simulink library "wnnmodels"  (R2021b)
settings: Solver=VariableStepAuto  StartTime=0.0  StopTime=10.0  RelTol=1e-3
undefined symbols (not defined in the file or in its folder): debug, mim_mem_size
libraries: simulink x2
settings Model: Creator=20214358  LastModifiedBy=20214358

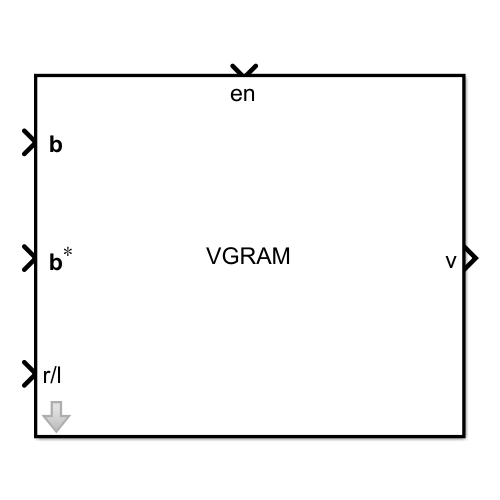
[thumbnail: Simulink's stored preview of the top-level diagram]
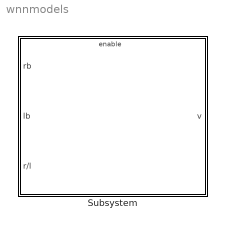
== system wnnmodels ==
  Subsystem : Subsystem  mask(Virtual Generalized Random Access Memory (VGRAM)){min_mem_size=[], max_mem_size=[], min_dist=[], max_dist=[]}
      mask prompts: min_mem_size "Minimum memory size"; max_mem_size "Maximum memory size"; min_dist "Minimum Hamming distance"; max_dist "Maximum Hamming distance"
      mask Display:
      | disp('VGRAM')
      | port_label('input', 1, '{\bf b}','interpreter','tex')
      | port_label('input', 2, '{\bf b}^{\ast}','interpreter','tex')
      | port_label('input', 3, 'r/l','interpreter','tex')
      | port_label('output', 1,'v','interpreter','tex')
      | port_label('Enable','en','interpreter','tex')

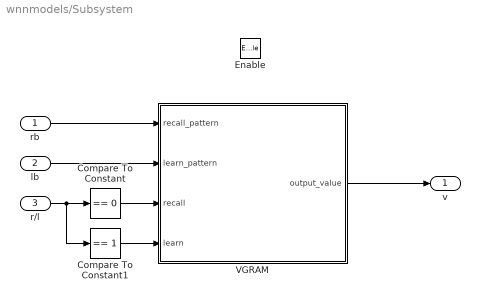
== system wnnmodels/Subsystem ==
  rb : Inport
  lb : Inport  Port=2
  r/l : Inport  Port=3
  Enable : EnablePort
  Compare To Constant : simulink/Logic and Bit Operations/Compare To Constant  relop===  const=0  OutDataTypeStr=boolean
  Compare To Constant1 : simulink/Logic and Bit Operations/Compare To Constant  relop===  const=1  OutDataTypeStr=boolean
  VGRAM : MATLAB Function  TreatAsAtomicUnit=on
  v : Outport
  wires:
  rb/1 -> VGRAM/1(recall_pattern)
  lb/1 -> VGRAM/2(learn_pattern)
  VGRAM/1(output_value) -> v/1
  r/l/1 -> Compare To Constant1/1, Compare To Constant/1
  Compare To Constant/1 -> VGRAM/3(recall)
  Compare To Constant1/1 -> VGRAM/4(learn)

== matlab function wnnmodels/Subsystem/VGRAM ==
  data: recall_pattern input; learn_pattern input; recall input; output_value output; learn input; mim_mem_size parameter; max_mem_size parameter; min_dist parameter; max_dist parameter; debug parameter
function output_value = fcn(recall_pattern, learn_pattern, recall, learn, mim_mem_size, max_mem_size, min_dist, max_dist, debug)

persistent input_patterns output_values valid_pairs num_valid_pairs last_output_value

pattern_length=length(recall_pattern);
if isempty(input_patterns)
    input_patterns = zeros(max_mem_size, pattern_length, 'logical');
    output_values = zeros(max_mem_size, 'uint64');
    valid_pairs = zeros(max_mem_size, 'logical');
    num_valid_pairs = uint32(0);
    last_output_value = uint64(0);
end

if(recall)
    % Default to zero
    output_value = uint64(0);

    if num_valid_pairs ~= uint32(0)
        % Filter out the valid input-output pairs
        valid_input_patterns = input_patterns(valid_pairs);
        valid_output_values = output_values(valid_pairs);

        aux = rand(num_valid_pairs,1);
    
        % Find the closest stored input pattern
        [closest_pattern_dist,closest_pattern_idx] = min(sum(bitxor(valid_input_patterns,recall_pattern),2)+aux);
        closest_pattern_dist = floor(closest_pattern_dist);
        
        if closest_pattern_dist <= max_dist
            % Return the output associated with the closest input pattern
            output_value = valid_output_values(closest_pattern_idx);
        end
    end

    % Save the last output value
    last_output_value = output_value;
end

if(learn)
    % Keep the last output value
    output_value = last_output_value;

    if num_valid_pairs == max_mem_size
        % Prune pairs low frequency pairs first

    end
    
    if num_valid_pairs == uint32(0)
        % Store the first input-output pair
        valid_pairs(1) = True;
        input_patterns(1) = learn_pattern;
        output_values(1) = uint64(1);
        num_valid_pairs = uint32(1);
    else
        aux = rand(max_mem_size,1);
        aux(valid_pairs) = Inf;

        % Find the closest stored input pattern
        [closest_pattern_dist,closest_pattern_idx] = min(sum(bitxor(input_patterns,recall_pattern),2)+aux);
        closest_pattern_dist = floor(closest_pattern_dist);  
        
        if closest_pattern_dist <= min_dist
            % Update an existing input-output pair
            output_values(closest_pattern_idx) = output_values(closest_pattern_idx) + uint64(1);
        else
            % Store a new input-output pair
            empty_entry_idx = find(~valid_pairs);
            valid_pairs(empty_entry_idx) = True;
            input_patterns(empty_entry_idx) = learn_pattern;
            output_values(empty_entry_idx) = uint64(1);
            num_valid_pairs = num_valid_pairs + uint32(1);
        end
    end    
end

if(debug)


end
